simulink model "temperature_change"  (R2024b)
settings: Solver=VariableStepAuto  StartTime=0.0  StopTime=10.0  RelTol=1e-3
settings Model: Creator=Amogh  LastModifiedBy=mr
settings ModelReferenceCC: EnableRefExpFcnMdlSchedulingChecks=on
settings RTWCC: GPUComputeCapability=3.5

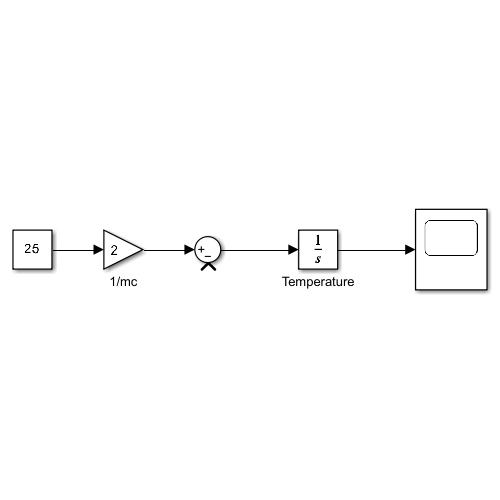
[thumbnail: Simulink's stored preview of the top-level diagram]
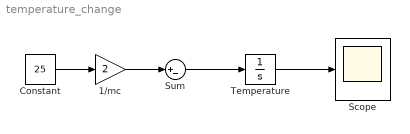
== system temperature_change ==
  1/mc : Gain  Gain=2
  Constant : Constant  Value=25
  Scope : Scope
  Sum : Sum  Inputs=|+-
  Temperature : Integrator
  wires:
  Constant/1 -> 1/mc/1
  Temperature/1 -> Scope/1
  1/mc/1 -> Sum/1
  Sum/1 -> Temperature/1
